simulink model "assignment_2_simulink"  (R2024a)
settings: Solver=ode23t  StartTime=0.0  StopTime=400  MaxStep=1e-4  RelTol=1e-3
values from neighbouring files (symbols this model uses):
  a = 0.5 * L    (= 1.385)    [assignment_2.m]
  Af = 2.37    [assignment_2.m]
  alpha_slope = 0    [assignment_2.m]
  b = 0.5 * L    (= 1.385)    [assignment_2.m]
  b_f = 0.75    [assignment_2.m]
  b_r = 1 - b_f    (= 0.25)    [assignment_2.m]
  bat_cap = 58000    [assignment_2.m]
  bat_per = 1    [assignment_2.m]
  Cx = 1    [assignment_2.m]
  drivetrain_gain = 10.5    [assignment_2.m]
  g = 9.81    [assignment_2.m]
  h = 0.55    [assignment_2.m]
  L = 2.77    [assignment_2.m]
  m = 1812    [assignment_2.m]
  R = 0.3488    [assignment_2.m]
  Rho = 0.27    [assignment_2.m]
  tau_b = 20*10^(-3)    (= 0.02)    [assignment_2.m]
  velstart = 20    [assignment_2.m]
settings Model: Creator=fjmo  LastModifiedBy=fjmo
settings SolverCC: AllowMultiTaskInputOutput=on
settings DebuggingCC: SignalInfNanChecking=error
settings ModelReferenceCC: ModelReferenceMinAlgLoopOccurrences=on

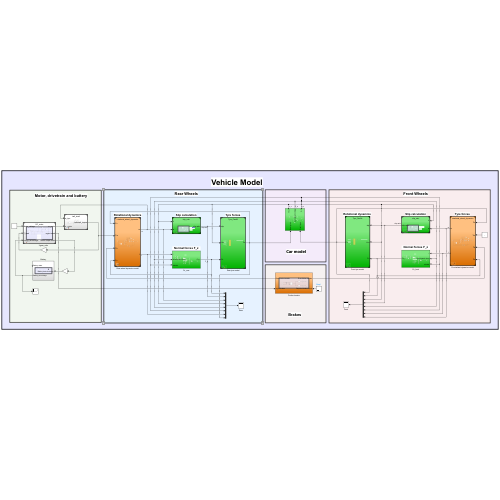
[thumbnail: Simulink's stored preview of the top-level diagram]
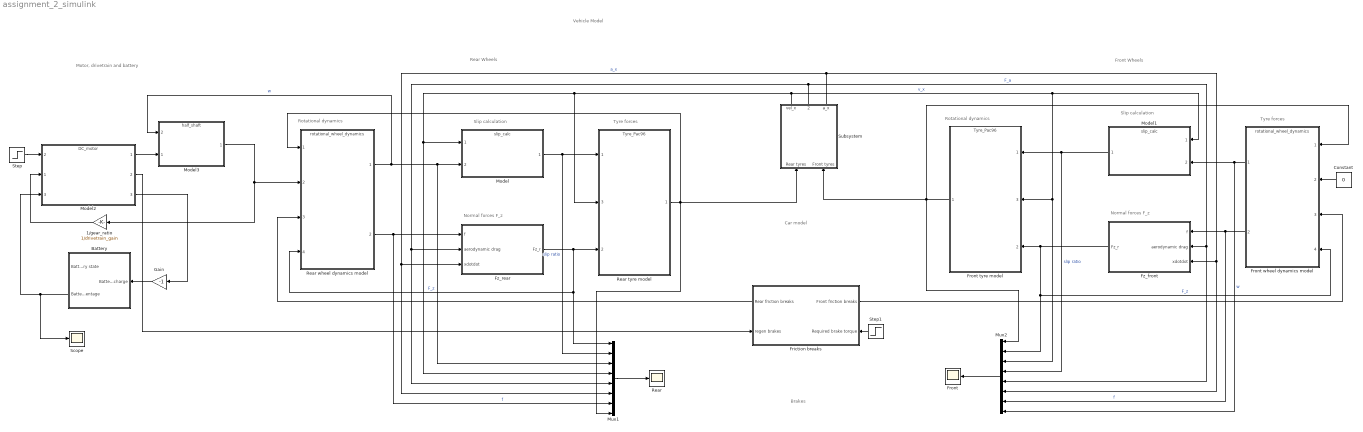
== system assignment_2_simulink ==
  note: Car model
  note: Brakes
  note: Rear Wheels
  note: Vehicle Model
  note: Slip calculation
  note: Rotational dynamics
  note: Normal forces F_z
  note: Tyre forces
  note: Normal forces F_z
  note: Slip calculation
  note: Tyre forces
  note: Rotational dynamics
  note: Front Wheels
  note: Motor, drivetrain and battery
  1/gear_ratio : Gain  Gain=1/drivetrain_gain
  Battery : Subsystem
  Constant : Constant  Value=0
  Friction breaks : Subsystem
      settings: PortSchema="{\"entries\":[{\"content\":{\"sides\":[{\"content\":{\"connectorIds\":[\"Out2\",\"In1\"]},\"type\":\"ConnectorPlacement.EquallySpacedRectSide\",\"uuid\":\"4a3dc718-d1bd-449b-9739-5f6ec97173fd\"},{\"content\":{\"connectorIds\":[\"Out1\",\"In2\"],\"side\":\"RIGHT\"},\"type\":\"ConnectorPlacement.EquallySpacedRectSide\",\"uuid\":\"f113ab5a-fdc2-44b8-a57e-3f1ebdb36388\"},{\"content\":{\"side\":\"TOP\"},\"type\":\"ConnectorPlacement.EquallySpacedRectSide\",\"uuid\":\"9daa155d-f8df-45ee-b4e4-423575000c04\"},{\"content\":{\"side\":\"BOTTOM\"},\"type\":\"ConnectorPlacement.EquallySpacedRectSide\",\"uuid\":\"a00ed6be-cc2c-4b97-89d3-ec6bcedf00be\"}]},\"type\":\"ConnectorPlacement.EquallySpacedConnector\",\"uuid\":\"52839571-6596-4419-b2fc-b5260a5b0043\"}],\"packageUris\":[\"http://schema.mathworks.com/mf0/Connector/R2020b\"],\"version\":\"1.0\"}"
  Front : Scope
  Front tyre model : ModelReference  ModelNameDialog=Tyre_Pac96.slx  SimulationMode=Normal  ModelReferenceVersion=9.38
      settings: PortSchema="{\"entries\":[{\"content\":{\"sides\":[{\"content\":{\"connectorIds\":[\"In2\",\"In3\",\"In1\"]},\"type\":\"ConnectorPlacement.EquallySpacedRectSide\",\"uuid\":\"128c3a03-d455-473f-b97a-1271ed5e183e\"},{\"content\":{\"connectorIds\":[\"Out1\"],\"side\":\"RIGHT\"},\"type\":\"ConnectorPlacement.EquallySpacedRectSide\",\"uuid\":\"90c93895-2958-47ec-b7e2-2fd8dd55f75c\"},{\"content\":{\"side\":\"TOP\"},\"type\":\"ConnectorPlacement.EquallySpacedRectSide\",\"uuid\":\"7d305e53-4902-4583-87fb-32e63dbec44e\"}]},\"type\":\"ConnectorPlacement.EquallySpacedConnector\",\"uuid\":\"7e04f67b-f04a-4aa3-857a-95fe89700190\"}],\"packageUris\":[\"http://schema.mathworks.com/mf0/Connector/R2020b\"],\"version\":\"1.0\"}"
  Front wheel dynamics model : ModelReference  ModelNameDialog=rotational_wheel_dynamics.slx  SimulationMode=Normal  ModelReferenceVersion=1.102
      settings: PortSchema="{\"entries\":[{\"content\":{\"sides\":[{\"content\":{\"connectorIds\":[\"In4\",\"In3\",\"In2\",\"In1\"]},\"type\":\"ConnectorPlacement.EquallySpacedRectSide\",\"uuid\":\"8e9cd13c-7748-4dfa-a955-38f4d392920c\"},{\"content\":{\"connectorIds\":[\"Out2\",\"Out1\"],\"side\":\"RIGHT\"},\"type\":\"ConnectorPlacement.EquallySpacedRectSide\",\"uuid\":\"81e5c474-d9e1-4061-825c-d1a8c8e14901\"},{\"content\":{\"side\":\"TOP\"},\"type\":\"ConnectorPlacement.EquallySpacedRectSide\",\"uuid\":\"fc221541-93a1-429d-a302-81ab5fdb9d5f\"}]},\"type\":\"ConnectorPlacement.EquallySpacedConnector\",\"uuid\":\"164d93d7-ac23-4763-b240-557da1fee494\"}],\"packageUris\":[\"http://schema.mathworks.com/mf0/Connector/R2020b\"],\"version\":\"1.0\"}"
  Fz_front : Subsystem
  Fz_rear : Subsystem
  Gain : Gain  Gain=-1
  Model : ModelReference  ModelNameDialog=slip_calc.slx  SimulationMode=Normal  ModelReferenceVersion=1.56
  Model1 : ModelReference  ModelNameDialog=slip_calc.slx  SimulationMode=Normal  ModelReferenceVersion=1.56
  Model2 : ModelReference  ModelNameDialog=DC_motor.slx  SimulationMode=Normal  ModelReferenceVersion=1.26
      settings: PortSchema="{\"entries\":[{\"content\":{\"sides\":[{\"content\":{\"connectorIds\":[\"In2\",\"In1\",\"In3\"]},\"type\":\"ConnectorPlacement.EquallySpacedRectSide\",\"uuid\":\"856ebdf3-b7b7-417f-9858-b4eab560afbe\"},{\"content\":{\"connectorIds\":[\"Out1\",\"Out2\",\"Out3\"],\"side\":\"RIGHT\"},\"type\":\"ConnectorPlacement.EquallySpacedRectSide\",\"uuid\":\"02573abb-4d18-4489-95c0-3c3e8424dddb\"},{\"content\":{\"side\":\"TOP\"},\"type\":\"ConnectorPlacement.EquallySpacedRectSide\",\"uuid\":\"d06d3c26-615d-4037-8c34-a23ff3cf08e1\"}]},\"type\":\"ConnectorPlacement.EquallySpacedConnector\",\"uuid\":\"1ed2590d-a287-4b16-8f7a-7838bb046942\"}],\"packageUris\":[\"http://schema.mathworks.com/mf0/Connector/R2020b\"],\"version\":\"1.0\"}"
  Model3 : ModelReference  ModelNameDialog=half_shaft.slx  SimulationMode=Normal  ModelReferenceVersion=1.9
      settings: PortSchema="{\"entries\":[{\"content\":{\"sides\":[{\"content\":{\"connectorIds\":[\"In2\",\"In1\"]},\"type\":\"ConnectorPlacement.EquallySpacedRectSide\",\"uuid\":\"2a87acde-a3e3-446f-b760-192272679fdf\"},{\"content\":{\"connectorIds\":[\"Out1\"],\"side\":\"RIGHT\"},\"type\":\"ConnectorPlacement.EquallySpacedRectSide\",\"uuid\":\"34dfae4c-dee8-4eab-a373-6b1516b3930c\"},{\"content\":{\"side\":\"TOP\"},\"type\":\"ConnectorPlacement.EquallySpacedRectSide\",\"uuid\":\"81d51af0-cac4-4152-bbe2-27ef4e77d1d7\"}]},\"type\":\"ConnectorPlacement.EquallySpacedConnector\",\"uuid\":\"9562c026-d786-4e9e-878e-61d7314473e4\"}],\"packageUris\":[\"http://schema.mathworks.com/mf0/Connector/R2020b\"],\"version\":\"1.0\"}"
  Mux1 : Mux  Inputs=8
  Mux2 : Mux  Inputs=8
  Rear : Scope
  Rear tyre model : ModelReference  ModelNameDialog=Tyre_Pac96.slx  SimulationMode=Normal  ModelReferenceVersion=9.38
      settings: PortSchema="{\"entries\":[{\"content\":{\"sides\":[{\"content\":{\"connectorIds\":[\"In1\",\"In3\",\"In2\"]},\"type\":\"ConnectorPlacement.EquallySpacedRectSide\",\"uuid\":\"128c3a03-d455-473f-b97a-1271ed5e183e\"},{\"content\":{\"connectorIds\":[\"Out1\"],\"side\":\"RIGHT\"},\"type\":\"ConnectorPlacement.EquallySpacedRectSide\",\"uuid\":\"90c93895-2958-47ec-b7e2-2fd8dd55f75c\"},{\"content\":{\"side\":\"TOP\"},\"type\":\"ConnectorPlacement.EquallySpacedRectSide\",\"uuid\":\"7d305e53-4902-4583-87fb-32e63dbec44e\"}]},\"type\":\"ConnectorPlacement.EquallySpacedConnector\",\"uuid\":\"7e04f67b-f04a-4aa3-857a-95fe89700190\"}],\"packageUris\":[\"http://schema.mathworks.com/mf0/Connector/R2020b\"],\"version\":\"1.0\"}"
  Rear wheel dynamics model : ModelReference  ModelNameDialog=rotational_wheel_dynamics.slx  SimulationMode=Normal  ModelReferenceVersion=1.102
  Scope : Scope
  Step : Step  Time=200  Before=400  After=0  SampleTime=0
  Step1 : Step  Time=200  After=200  SampleTime=0
  Subsystem : Subsystem
  wires:
  Subsystem/2(aerodynamic drag) -> Fz_rear/2(aerodynamic drag), Mux1/5, Fz_front/2(aerodynamic drag), Mux2/5  "F_a"
  Fz_rear/1(Fz_r) -> Rear tyre model/2, Mux1/1, Rear wheel dynamics model/4  "F_z"
  Model/1 -> Rear tyre model/1, Mux1/2  "slip ratio"
  Rear wheel dynamics model/1 -> Model3/2, Model/2, Mux1/3  "w"
  Subsystem/3(a_x) -> Mux1/6, Fz_rear/3(xdotdot), Mux2/6, Fz_front/3(xdotdot)  "a_x"
  Rear tyre model/1 -> Subsystem/1(Rear tyres), Mux1/8, Rear wheel dynamics model/1
  Rear wheel dynamics model/2 -> Fz_rear/1(f), Mux1/7  "f"
  Subsystem/1(vel_x) -> Rear tyre model/3, Mux1/4, Model/1, Model1/1, Mux2/3, Front tyre model/3  "v_x"
  Front wheel dynamics model/2 -> Fz_front/1(f), Mux2/7  "f"
  Front wheel dynamics model/1 -> Model1/2, Mux2/8  "w"
  Mux2/1 -> Front/1
  Fz_front/1(Fz_r) -> Mux2/2, Front wheel dynamics model/4, Front tyre model/2  "F_z"
  Model1/1 -> Front tyre model/1, Mux2/4  "slip ratio"
  Front tyre model/1 -> Mux2/1, Front wheel dynamics model/1, Subsystem/2(Front tyres)
  Mux1/1 -> Rear/1
  Constant/1 -> Front wheel dynamics model/2
  Friction breaks/1(Front friction breaks) -> Front wheel dynamics model/3
  Model2/1 -> Model3/1
  1/gear_ratio/1 -> Model2/1
  Step/1 -> Model2/2
  Model3/1 -> Rear wheel dynamics model/2, 1/gear_ratio/1
  Friction breaks/2(Rear friction breaks) -> Rear wheel dynamics model/3
  Model2/2 -> Friction breaks/1(regen brakes)
  Battery/2(Battery percentage) -> Scope/1, Model2/3
  Step1/1 -> Friction breaks/2(Required brake torque)
  Gain/1 -> Battery/1(Battery drain/recharge)
  Model2/3 -> Gain/1

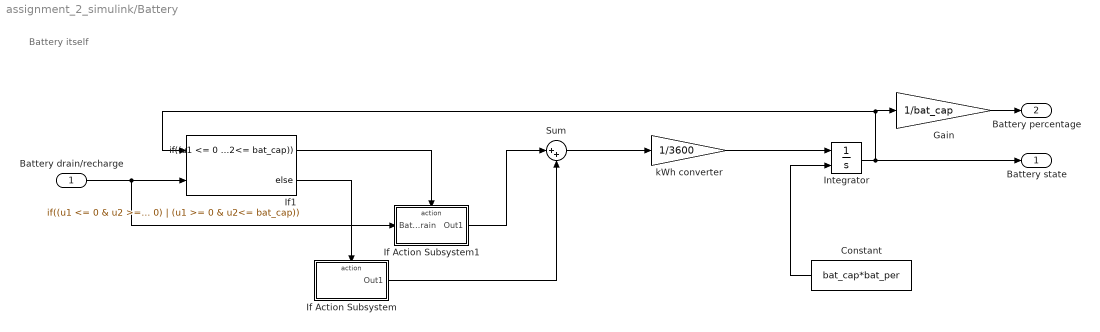
== system assignment_2_simulink/Battery ==
  note: Battery itself
  Battery drain/recharge : Inport
  Constant : Constant  Value=bat_cap*bat_per
  Gain : Gain  Gain=1/bat_cap
  If Action Subsystem : Subsystem  TreatAsAtomicUnit=on
  If Action Subsystem1 : Subsystem  TreatAsAtomicUnit=on
  If1 : If  NumInputs=2  IfExpression=(u1 <= 0 & u2 >= 0) | (u1 >= 0 & u2<= bat_cap)
  Integrator : Integrator  InitialConditionSource=external
  Sum : Sum  Inputs=|++
  kWh converter : Gain  Gain=1/3600
  Battery state : Outport
  Battery percentage : Outport  Port=2
  wires:
  Constant/1 -> Integrator/2
  Integrator/1 -> Battery state/1, Gain/1, If1/1
  Gain/1 -> Battery percentage/1
  kWh converter/1 -> Integrator/1
  Sum/1 -> kWh converter/1
  Battery drain/recharge/1 -> If Action Subsystem1/1(Battery charge/drain), If1/2
  If1/2 -> If Action Subsystem/Action
  If1/1 -> If Action Subsystem1/Action
  If Action Subsystem1/1(Out1) -> Sum/1
  If Action Subsystem/1(Out1) -> Sum/2

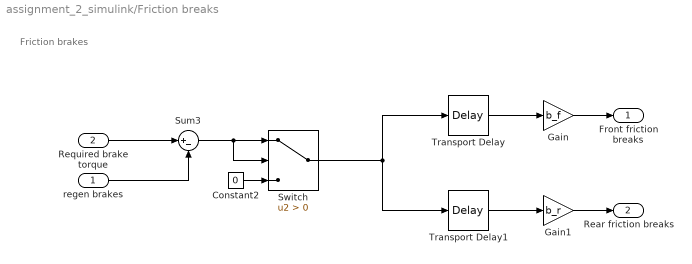
== system assignment_2_simulink/Friction breaks ==
  note: Friction brakes
  regen brakes : Inport
  Required brake torque : Inport  Port=2
  Constant2 : Constant  Value=0
  Gain : Gain  Gain=b_f
  Gain1 : Gain  Gain=b_r
  Sum3 : Sum  Inputs=|+-
  Switch : Switch  Criteria=u2 > Threshold  SaturateOnIntegerOverflow=off  InputSameDT=off
  Transport Delay : TransportDelay  DelayTime=tau_b
  Transport Delay1 : TransportDelay  DelayTime=tau_b
  Front friction breaks : Outport
  Rear friction breaks : Outport  Port=2
  wires:
  Gain/1 -> Front friction breaks/1
  Gain1/1 -> Rear friction breaks/1
  Transport Delay/1 -> Gain/1
  Transport Delay1/1 -> Gain1/1
  Switch/1 -> Transport Delay/1, Transport Delay1/1
  Required brake torque/1 -> Sum3/1
  regen brakes/1 -> Sum3/2
  Sum3/1 -> Switch/2, Switch/1
  Constant2/1 -> Switch/3

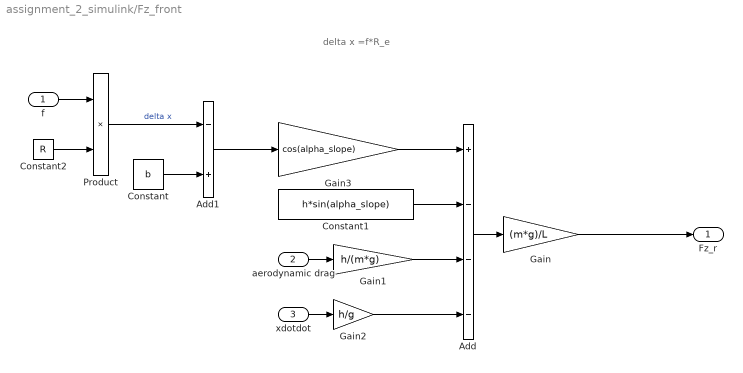
== system assignment_2_simulink/Fz_front ==
  note: delta x =f*R_e
  f : Inport
  aerodynamic drag : Inport  Port=2
  xdotdot : Inport  Port=3
  Add : Sum  Inputs=+---
  Add1 : Sum  Inputs=-+
  Constant : Constant  Value=b
  Constant1 : Constant  Value=h*sin(alpha_slope)
  Constant2 : Constant  Value=R
  Gain : Gain  Gain=(m*g)/L
  Gain1 : Gain  Gain=h/(m*g)
  Gain2 : Gain  Gain=h/g
  Gain3 : Gain  Gain=cos(alpha_slope)
  Product : Product
  Fz_r : Outport
  wires:
  aerodynamic drag/1 -> Gain1/1
  Gain3/1 -> Add/1
  Constant1/1 -> Add/2
  Gain1/1 -> Add/3
  Gain2/1 -> Add/4
  xdotdot/1 -> Gain2/1
  Add/1 -> Gain/1
  Product/1 -> Add1/1  "delta x"
  Constant/1 -> Add1/2
  Add1/1 -> Gain3/1
  f/1 -> Product/1
  Constant2/1 -> Product/2
  Gain/1 -> Fz_r/1

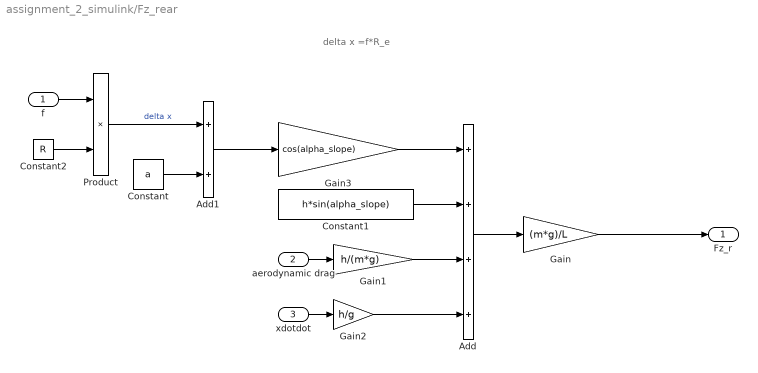
== system assignment_2_simulink/Fz_rear ==
  note: delta x =f*R_e
  f : Inport
  aerodynamic drag : Inport  Port=2
  xdotdot : Inport  Port=3
  Add : Sum  Inputs=++++
  Add1 : Sum
  Constant : Constant  Value=a
  Constant1 : Constant  Value=h*sin(alpha_slope)
  Constant2 : Constant  Value=R
  Gain : Gain  Gain=(m*g)/L
  Gain1 : Gain  Gain=h/(m*g)
  Gain2 : Gain  Gain=h/g
  Gain3 : Gain  Gain=cos(alpha_slope)
  Product : Product
  Fz_r : Outport
  wires:
  aerodynamic drag/1 -> Gain1/1
  Gain3/1 -> Add/1
  Constant1/1 -> Add/2
  Gain1/1 -> Add/3
  Gain2/1 -> Add/4
  xdotdot/1 -> Gain2/1
  Add/1 -> Gain/1
  Product/1 -> Add1/1  "delta x"
  Constant/1 -> Add1/2
  Add1/1 -> Gain3/1
  f/1 -> Product/1
  Constant2/1 -> Product/2
  Gain/1 -> Fz_r/1

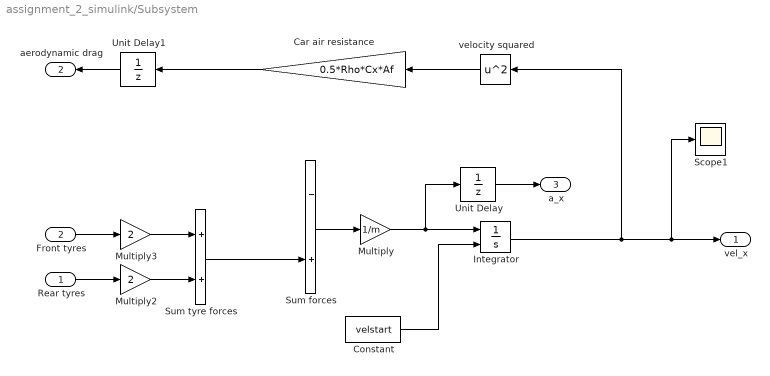
== system assignment_2_simulink/Subsystem ==
  Rear tyres : Inport
  Front tyres : Inport  Port=2
  Car air resistance : Gain  Gain=0.5*Rho*Cx*Af
  Constant : Constant  Value=velstart
  Integrator : Integrator  InitialConditionSource=external
  Multiply : Gain  Gain=1/m
  Multiply2 : Gain  Gain=2
  Multiply3 : Gain  Gain=2
  Scope1 : Scope
  Sum forces : Sum  Inputs=-+
  Sum tyre forces : Sum
  Unit Delay : UnitDelay  SampleTime=-1  HasFrameUpgradeWarning=on
  Unit Delay1 : UnitDelay  SampleTime=-1  HasFrameUpgradeWarning=on
  velocity squared : Math  Operator=square  SignedPower=on  RndMeth=Zero
  vel_x : Outport
  aerodynamic drag : Outport  Port=2
  a_x : Outport  Port=3
  wires:
  Sum forces/1 -> Multiply/1
  Sum tyre forces/1 -> Sum forces/2
  velocity squared/1 -> Car air resistance/1
  Constant/1 -> Integrator/2
  Integrator/1 -> vel_x/1, Scope1/1, velocity squared/1
  Front tyres/1 -> Multiply3/1
  Rear tyres/1 -> Multiply2/1
  Multiply2/1 -> Sum tyre forces/2
  Multiply3/1 -> Sum tyre forces/1
  Multiply/1 -> Unit Delay/1, Integrator/1
  Car air resistance/1 -> Unit Delay1/1
  Unit Delay/1 -> a_x/1
  Unit Delay1/1 -> aerodynamic drag/1

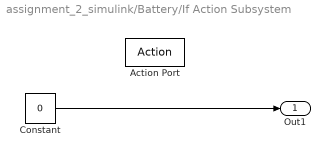
== system assignment_2_simulink/Battery/If Action Subsystem ==
  Action Port : ActionPort  ActionPortLabel=else
  Constant : Constant  Value=0
  Out1 : Outport
  wires:
  Constant/1 -> Out1/1

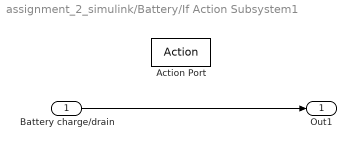
== system assignment_2_simulink/Battery/If Action Subsystem1 ==
  Battery charge/drain : Inport
  Action Port : ActionPort  ActionPortLabel=if((u1 <= 0 & u2 >= 0) | (u1 >= 0 & u2<= bat_cap))
  Out1 : Outport
  wires:
  Battery charge/drain/1 -> Out1/1
